simulink model "mc1_openloop"  (R2023b)
settings: Solver=ode45  StartTime=0.0  StopTime=8.0  MaxStep=1e-5  RelTol=1e-3
libraries: spsDCVoltageSourceLib x1, simulink x1, spsUniversalBridgeLib x1, spsVoltageMeasurementLib x1, spspowerguiLib x1
settings Model: Creator=86189  LastModifiedBy=86189

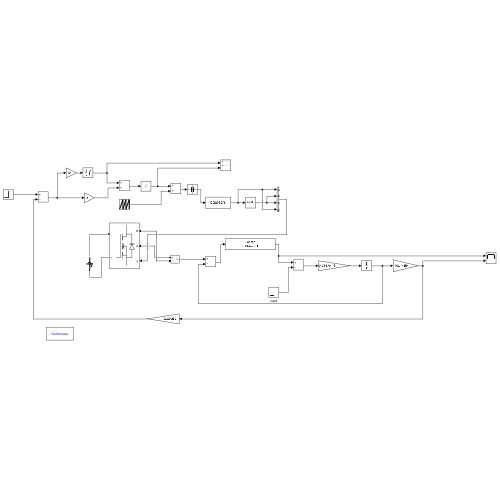
[thumbnail: Simulink's stored preview of the top-level diagram]
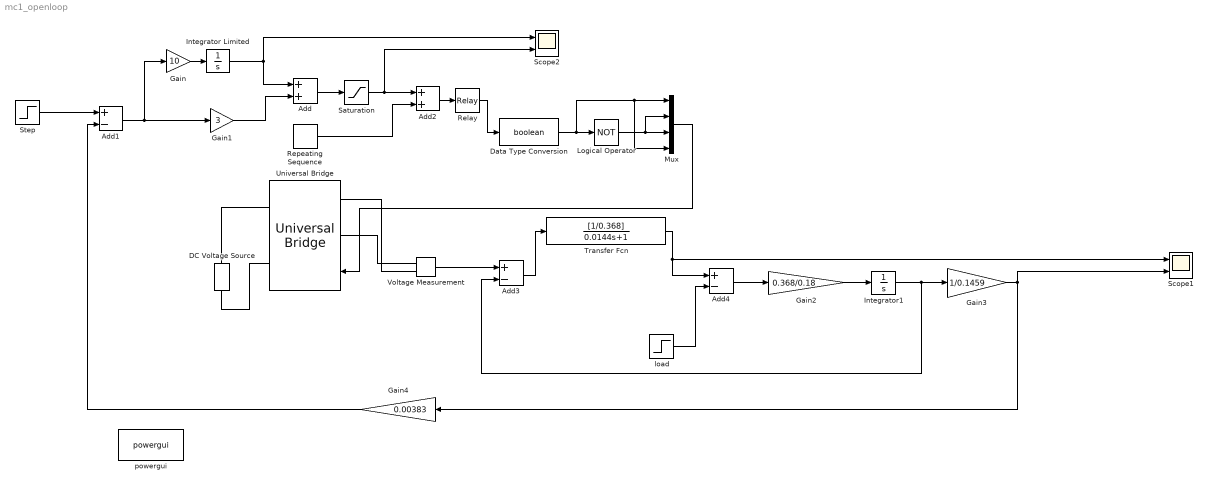
== system mc1_openloop ==
  Add : Sum
  Add1 : Sum  Inputs=+-
  Add2 : Sum
  Add3 : Sum  Inputs=+-
  Add4 : Sum  Inputs=+-
  DC Voltage Source : spsDCVoltageSourceLib/DC Voltage Source  Amplitude=538  Measurements=None
  Data Type Conversion : DataTypeConversion  OutDataTypeStr=boolean  SaturateOnIntegerOverflow=off  RndMeth=Floor
  Gain : Gain  Gain=10
  Gain1 : Gain  Gain=3
  Gain2 : Gain  Gain=0.368/0.18
  Gain3 : Gain  Gain=1/0.1459
  Gain4 : Gain  Gain=0.00383
  Integrator Limited : Integrator  LimitOutput=on  UpperSaturationLimit=5  LowerSaturationLimit=-5
  Integrator1 : Integrator
  Logical Operator : Logic  Operator=NOT  AllPortsSameDT=off  OutDataTypeStr=boolean
  Mux : Mux
      settings: DisplayOption=signals
  Relay : Relay  OnSwitchValue=0  OffSwitchValue=0
  Repeating Sequence : simulink/Sources/Repeating Sequence  rep_seq_t=[0 0.125e-3]  rep_seq_y=[-5 5]
  Saturation : Saturate  UpperLimit=5  LowerLimit=-5
  Scope1 : Scope  NumInputPorts=2
  Scope2 : Scope  NumInputPorts=2
  Step : Step  Time=0  After=10  SampleTime=0
  Transfer Fcn : TransferFcn  Numerator=[1/0.368]  Denominator=[0.0144 1]
  Universal Bridge : spsUniversalBridgeLib/Universal Bridge  Arms=2  SnubberResistance=1e5  SnubberCapacitance=inf  Device=MOSFET / Diodes  Ron=1e-3  Lon=0  ForwardVoltages="[  0  0  ]"  ForwardVoltage=0  GTOparameters=[ 10e-6 , 20e-6 ]  IGBTparameters=[ 1e-6 , 2e-6 ]  Measurements=None  Measurements_2=None  converterType=Rectifier
  Voltage Measurement : spsVoltageMeasurementLib/Voltage Measurement  PhasorSimulation=off  OutputType=Complex  PSBequivalent=0
  load : Step  Time=0  After=10  SampleTime=0
  powergui : spspowerguiLib/powergui  Priority=1  SimulationMode=Continuous  SampleTime=50e-6  frequency=60  Iterations=50  frequencyindice=0  Pbase=100e6  ErrMax=1e-4  UnitsV=kV  UnitsW=MW  buscounter=0  FunctionMessages=off  echomessages=off  EnableUseOfTLC=off  CurrentSourceSwitches=off  DisableSnubberDevices=off  DisableRonSwitches=off  DisableVfSwitches=off  DisplayEquations=off  AutomaticDiscreteSolvers=off  SolverType=Tustin/Backward Euler (TBE)  Interpol=off  ExternalGateDelay=off  methode=off  Ts=100  x0status=blocks  SPID=on  SwTol=0  HookPort=off  NonlinearTolerance=1e-4  nMaxIteration=100  ContinueOnMaxIteration=off  RestoreLinks=warning  ResistiveCurrentMeasurement=off  Frange=[0:2:500]  Ylog=off  Xlog=on  ShowGrid=off  save=off  variable=ZData  structure=0  ZoomFFT=off  StartTime=0.0  cycles=1  DisplayStyle=1  fundamental=60  FreqAxis=off  MaxFrequency=1000  frequencyindicesteady=1  RmsSteady=1  display=off
  wires:
  Integrator Limited/1 -> Scope2/1, Add/1
  Gain/1 -> Integrator Limited/1
  Add1/1 -> Gain/1, Gain1/1
  Saturation/1 -> Scope2/2, Add2/1
  Repeating Sequence/1 -> Add2/2
  Add2/1 -> Relay/1
  Mux/1 -> Universal Bridge/1
  Voltage Measurement/1 -> Add3/1
  Add3/1 -> Transfer Fcn/1
  load/1 -> Add4/2
  Add4/1 -> Gain2/1
  Gain2/1 -> Integrator1/1
  Integrator1/1 -> Add3/2, Gain3/1
  Transfer Fcn/1 -> Add4/1, Scope1/1
  Gain4/1 -> Add1/2
  Gain3/1 -> Gain4/1, Scope1/2
  Relay/1 -> Data Type Conversion/1
  Data Type Conversion/1 -> Mux/4, Mux/1, Logical Operator/1
  Logical Operator/1 -> Mux/2, Mux/3
  Step/1 -> Add1/1
  Gain1/1 -> Add/2
  Add/1 -> Saturation/1
  connections:
  Universal Bridge/LConn1 -- Voltage Measurement/LConn1
  Universal Bridge/LConn2 -- Voltage Measurement/LConn2
  DC Voltage Source/RConn1 -- Universal Bridge/RConn1
  Universal Bridge/RConn2 -- DC Voltage Source/LConn1
